simulink model "spacecraft4_2"  (R2019b)
settings: Solver=VariableStepAuto  StartTime=0.0  StopTime=10.0  RelTol=1e-3
values from neighbouring files (symbols this model uses):
  K = lqr(A,B,Q,R)    [LQG_calcs.m]
  R = 0.001    [LQG_calcs.m]
  sysKF = ss(A-Kf*C,[B Kf],eye(3),0*[B Kf])    [LQG_calcs.m]
undefined symbols (not defined in the file or in its folder): Discrete, Time
libraries: ctrlSharedLib x1
settings Model: Creator=Tesla  LastModifiedBy=Tesla

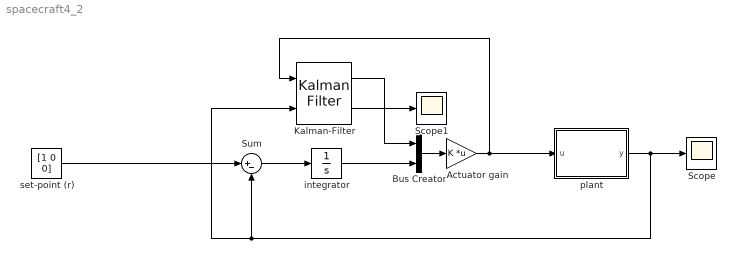
== system spacecraft4_2 ==
  Actuator gain : Gain  Gain=K  Multiplication=Matrix(K*u) (u vector)
  Bus Creator : BusCreator  Inputs=2
  Kalman-Filter : ctrlSharedLib/Kalman Filter  TimeDomain=Discrete-Time  UseCurrentEstimator=on  ModelSource=Individual A, B, C, D matrices  ModelSourceVariable=ss(0.95,1,1,0,1)  A=sysKF.A  B=sysKF.B  C=sysKF.C  D=sysKF.D  NumberOfStates=1  NumberOfInputs=1  NumberOfOutputs=1  InitialEstimateSource=Dialog  X0=0  P0=10  UseK=off  UseGH=off  NumberOfProcessNoiseInputs=1  G=1  TimeInvariantG=on  H=0  TimeInvariantH=on  Q=Q  TimeInvariantQ=on  R=R  TimeInvariantR=on  N=0  TimeInvariantN=on  AddInputPort=on  AddEnablePort=off  OutputEstimatedY=on  OutputP=off  Ts=-1
      settings: SourceProductBaseCode=CT
  Scope : Scope
  Scope1 : Scope
  Sum : Sum  Inputs=|+-
  integrator : Integrator
  "plant " : MATLAB Function  TreatAsAtomicUnit=on
  set-point (r) : Constant  Value=[1 0 0]
  wires:
  "plant "/1(y) -> Scope/1, Kalman-Filter/2, Sum/2
  Sum/1 -> integrator/1
  Actuator gain/1 -> "plant "/1(u), Kalman-Filter/1
  Kalman-Filter/1 -> Bus Creator/1
  Bus Creator/1 -> Actuator gain/1
  integrator/1 -> Bus Creator/2
  Kalman-Filter/2 -> Scope1/1
  set-point (r)/1 -> Sum/1

== matlab function spacecraft4_2/plant  ==
  data: u input; y output
function y = fcn(u)


y = 0.2*u;
